simulink model "ModeloLabo2"  (R2026a)
settings: Solver=VariableStepAuto
values from neighbouring files (symbols this model uses):
  Kc = (tao + tdead/2) / (Kp * (tauc + tdead/2))    (= 4.19621754571)    [FiguraModeloH.m]    (also in FiguraModeloMoro.m = 3.72180310381; FigureHPerturbacion.m; FigureMoroPerturbacion.m = 3.72180310381; ModeloLabo2H.m)
  Td = (tao * tdead) / (2 * tao + tdead)    (= 18.7462883489)    [FiguraModeloH.m]    (also in FiguraModeloMoro.m = 8.78829; FiguraModeloTurner.m = 0; FiguraTurnerPerturbacion.m = 0; FigureHPerturbacion.m)
  tesc = 5    [CodigoTurner.m]    (also in CodigoTurnerPerturbacion.m; FiguraModeloH.m; FiguraModeloMoro.m; FiguraModeloTurner.m)
  Ti = tao + tdead/2    (= 201.0065)    [FiguraModeloH.m]    (also in FiguraModeloMoro.m = 150.6564; FiguraModeloTurner.m = 117.025209274; FiguraTurnerPerturbacion.m = 117.025209274; FigureHPerturbacion.m)
libraries: realtime_pacer_lib x1
settings Model: Creator=Nehir RT  LastModifiedBy=Nehir RT

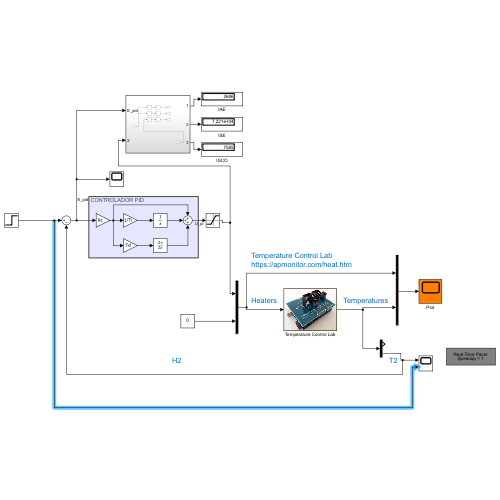
[thumbnail: Simulink's stored preview of the top-level diagram]
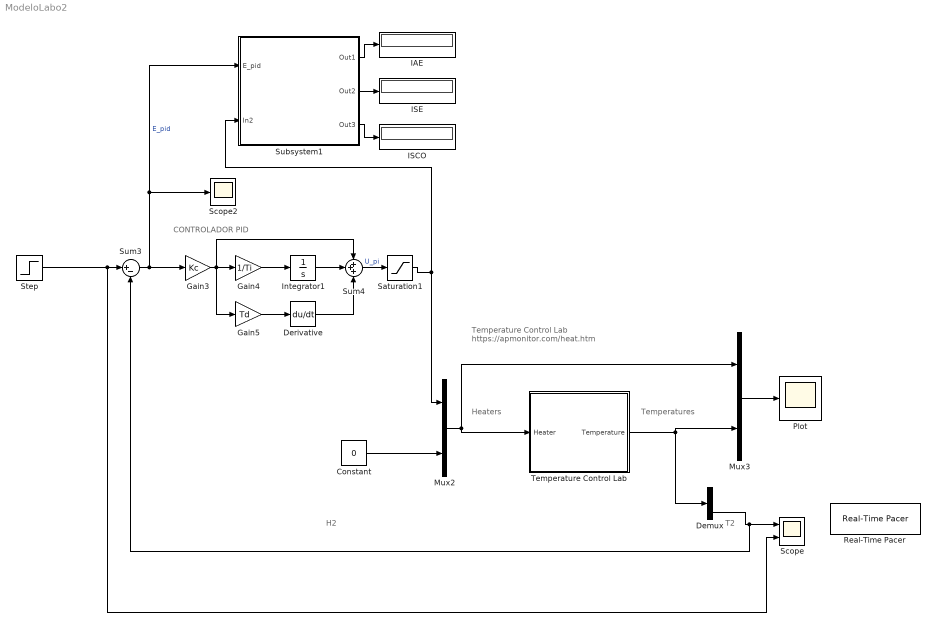
== system ModeloLabo2 ==
  note: Temperature Control Lab
      | https://apmonitor.com/heat.htm
  note: Temperatures
  note: H2
  note: Heaters
  note: T2
  note: CONTROLADOR PID
  Constant : Constant  Value=0
  Demux : Demux  Outputs=2
  Derivative : Derivative
  Gain3 : Gain  Gain=Kc
  Gain4 : Gain  Gain=1/Ti
  Gain5 : Gain  Gain=Td
  IAE : Display
  ISCO : Display
  ISE : Display
  Integrator1 : Integrator
  Mux2 : Mux  Inputs=2
  Mux3 : Mux  Inputs=2
  Plot : Scope
      settings: ActiveDisplayYMinimum=-32.084528563374562  ActiveDisplayYMaximum=117.69976824260141  DataLoggingSaveFormat=Array
  Real-Time Pacer : realtime_pacer_lib/Real-Time Pacer  simTimePerRealTime=1
      settings: SourceProductName=Real-Time Pacer
  Saturation1 : Saturate  UpperLimit=100  LowerLimit=0
  Scope : Scope  NumInputPorts=2
      settings: ActiveDisplayYMinimum=-6.4999999999999982  ActiveDisplayYMaximum=58.5  DataLoggingVariableName=DatosOut
  Scope2 : Scope
      settings: ActiveDisplayYMinimum=-1  ActiveDisplayYMaximum=1  DataLoggingVariableName=ScopeData2
  Step : Step  Time=tesc  FinalValue=Aesc  SampleTime=0
  Subsystem1 : Subsystem
  Sum3 : Sum  Inputs=|+-
  Sum4 : Sum  Inputs=+++
  Temperature Control Lab : Subsystem
      mask Display: image('tclab.png');
  wires:
  Mux3/1 -> Plot/1
  Demux/2 -> Sum3/2, Scope/1
  Mux2/1 -> Mux3/1, Temperature Control Lab/1(Heater)
  Step/1 -> Sum3/1, Scope/2
  Temperature Control Lab/1(Temperature) -> Mux3/2, Demux/1
  Constant/1 -> Mux2/2
  Saturation1/1 -> Mux2/1, Subsystem1/2(In2)
  Gain4/1 -> Integrator1/1
  Subsystem1/2(Out2) -> ISE/1
  Sum4/1 -> Saturation1/1  "U_pi"
  Subsystem1/3(Out3) -> ISCO/1
  Gain5/1 -> Derivative/1
  Sum3/1 -> Gain3/1, Subsystem1/1(E_pid), Scope2/1  "E_pid"
  Integrator1/1 -> Sum4/2
  Gain3/1 -> Gain5/1, Gain4/1, Sum4/1
  Subsystem1/1(Out1) -> IAE/1
  Derivative/1 -> Sum4/3

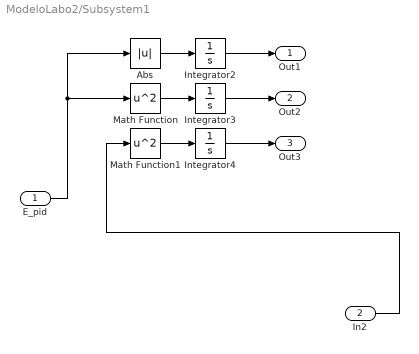
== system ModeloLabo2/Subsystem1 ==
  E_pid : Inport
  In2 : Inport  Port=2
  Abs : Abs  SaturateOnIntegerOverflow=off
  Integrator2 : Integrator
  Integrator3 : Integrator
  Integrator4 : Integrator
  Math Function : Math  Operator=square
  Math Function1 : Math  Operator=square
  Out1 : Outport
  Out2 : Outport  Port=2
  Out3 : Outport  Port=3
  wires:
  E_pid/1 -> Math Function/1, Abs/1
  Math Function/1 -> Integrator3/1
  Integrator4/1 -> Out3/1
  Abs/1 -> Integrator2/1
  Math Function1/1 -> Integrator4/1
  Integrator3/1 -> Out2/1
  In2/1 -> Math Function1/1
  Integrator2/1 -> Out1/1

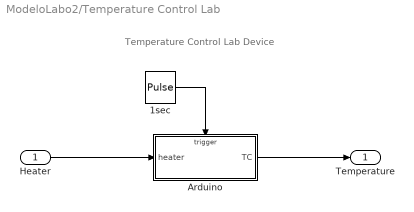
== system ModeloLabo2/Temperature Control Lab ==
  note: Temperature Control Lab Device
  Heater : Inport
  1sec : DiscretePulseGenerator  PulseType=Time based  Period=1  PulseWidth=50
  Arduino : Subsystem  TreatAsAtomicUnit=on
  Temperature : Outport  VectorParamsAs1DForOutWhenUnconnected=off
  wires:
  1sec/1 -> Arduino/Trigger
  Arduino/1(TC) -> Temperature/1
  Heater/1 -> Arduino/1(heater)

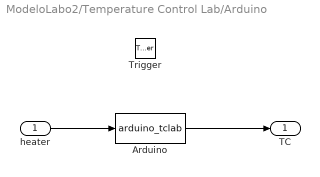
== system ModeloLabo2/Temperature Control Lab/Arduino ==
  heater : Inport  LatchByDelayingOutsideSignal=on
  Trigger : TriggerPort  VariantControl=Variant
  Arduino : MATLABFcn  MATLABFcn=arduino_tclab
  TC : Outport  InitialOutput=[23 23]  VectorParamsAs1DForOutWhenUnconnected=off
  wires:
  heater/1 -> Arduino/1
  Arduino/1 -> TC/1
